simulink model "Non_WindFarm"  (R2024a)
settings: Solver=ode45  StartTime=parSimulacio.ti  StopTime=200  MaxStep=parSimulacio.pas  RelTol=1e-6  AbsTol=1e-6  EnableMultiTasking=on
model workspace (MAT data in the model file):
  tt_vw : Simulink.Parameter (value not decoded)
values from neighbouring files (symbols this model uses):
  L = L'    [Lin_SignalGenerator.m]    (also in Non_ParameterInitialize.m; cal_QR.m = zeros(v, 1); parameters_windFarm2.m)
  nu = size(S, 1)    [Lin_SignalGenerator.m]    (also in Non_ParameterInitialize.m; parameters_windFarm2.m)
  S = zeros(v, v)    [cal_QR.m]
  w0 = [1 -0.00962521549583 0.0254779042049 -0.0160197396127 -0.0156056332727 0.0112137208272 0.0440607583301 -0.0193704893312 -0.0229464276306 -0.00247675309015 0.0285830611299]    [w0.mat]
undefined symbols (not defined in the file or in its folder): parControl, parConvertidor, parGenerador, parGrid, parMecanica, parSimulacio, windspeed
(part 28 of 40)

== system Non_WindFarm/FOM/Wind Farm/Wind Turbine Strings/String6/WT9/WFG/Maquina Sincrona ==
  note: Eq 4.22
  note: park transformation & Inverse
  note: theta_r
  note: Electrical angle=Mechnical angle *Pole Pairs
  note: Omega_r=Omega_m*P
  vsabc : Inport
  omega_m : Inport  Port=2
  theta_m : Inport  Port=3  PortDimensions=1
  Add : Sum  Inputs=+++
  Constant : Constant  Value=-rs/Lq
  Constant1 : Constant  Value=-rs/Ld
  Constant2 : Constant  Value=[1/Lq;0]
  Constant3 : Constant  Value=[1/Lq,0;0,1/Ld]
  Demux : Demux  Outputs=2
  Gain : Gain  Gain=-Ld/Lq
  Gain1 : Gain  Gain=Lq/Ld
  Gain2 : Gain  Gain=-lambda_m
  Gain3 : Gain  Gain=lambda_m
  Gain4 : Gain  Gain=Ld-Lq
  Gain5 : Gain  Gain=3/2*P
  Gain6 : Gain  Gain=P
  Gain7 : Gain  Gain=P
  Integrator : Integrator  InitialCondition=isqd0
  Matrix Concatenate : Concatenate  Mode=Multidimensional array  ConcatenateDimension=2
  Mux : Mux  Inputs=2
  Mux1 : Mux  Inputs=2
  Park : Subsystem
  Product{,2,4..5} (4 alike) : Product  Multiplication=Matrix(*)  RndMeth=Zero
  Product1 : Product  RndMeth=Zero
  Product3 : Product  RndMeth=Zero
  Sum : Sum  Inputs=|++
  isabc : Outport
  parell_m : Outport  Port=2
  wires:
  Constant/1 -> Mux/1
  Gain1/1 -> Mux/2
  Gain/1 -> Mux1/1
  Constant1/1 -> Mux1/2
  omega_m/1 -> Gain6/1
  Mux/1 -> Matrix Concatenate/1
  Mux1/1 -> Matrix Concatenate/2
  Matrix Concatenate/1 -> Product/1
  Product/1 -> Add/1
  Add/1 -> Integrator/1  "disqd"
  Integrator/1 -> Demux/1, Product5/2, Product/2  "isqd"
  Gain2/1 -> Product1/2
  Constant2/1 -> Product1/1
  Product1/1 -> Add/2
  Constant3/1 -> Product2/1
  Product2/1 -> Add/3
  Demux/1 -> Gain3/1, Product3/2
  Product3/1 -> Gain4/1
  Demux/2 -> Product3/1
  Gain3/1 -> Sum/1
  Gain4/1 -> Sum/2
  Sum/1 -> Gain5/1
  Gain5/1 -> parell_m/1
  Gain6/1 -> Gain1/1, Gain/1, Gain2/1
  theta_m/1 -> Gain7/1
  Product4/1 -> Product2/2
  Park/1(Tthetar) -> Product4/1
  Gain7/1 -> Park/1(theta_r)
  Park/2(nTthetar) -> Product5/1
  Product5/1 -> isabc/1
  vsabc/1 -> Product4/2

== system Non_WindFarm/FOM/Wind Farm/Wind Turbine Strings/String6/WT9/WFG/Mecanica nolineal i vent ==
  note: gearbox ration
  note: Gamma_t
  parell_m : Inport
  theta_a : Inport  Port=2
  vw : Inport  Port=3
  Gain1 : Gain  Gain=1/It
  Gain2 : Gain  Gain=nu
  Gain4 : Gain  Gain=nu
  Gain5 : Gain  Gain=nu
  Integrator : Integrator  InitialCondition=omegat0
  Integrator1 : Integrator
  Saturation : Saturate  UpperLimit=inf  LowerLimit=1e-6
  Sum : Sum  Inputs=++|
  Transfer Fcn : TransferFcn  Denominator=[taupitch 1]
  Turbina : Subsystem  mask{rho=1.225, R=R, cs=[0.5 116 0.4 0 0 5 21 0.08 0.035]}
      mask prompts: rho "Densitat de l'aire (Kg/m^3)"; R "Radi (R)"; cs "Constants [c1 c2 .. c9]"
      mask init:
      | A=pi*R^2;
      | c1=cs(1);
      | c2=cs(2);
      | c3=cs(3);
      | c4=cs(4);
      | c5=cs(5);
      | c6=cs(6);
      | c7=cs(7);
      | c8=cs(8);
      | c9=cs(9);
  omega_m : Outport
  theta_m : Outport  Port=2
  Cp : Outport  Port=3
  theta_aleps : Outport  Port=4
  wires:
  Sum/1 -> Gain1/1
  Gain1/1 -> Integrator/1
  Integrator/1 -> Integrator1/1, Gain4/1, Saturation/1
  Turbina/1(parell_turbina) -> Sum/2
  Gain2/1 -> Sum/1
  parell_m/1 -> Gain2/1
  Integrator1/1 -> Gain5/1
  Gain4/1 -> omega_m/1
  Gain5/1 -> theta_m/1
  Saturation/1 -> Turbina/2(omega_aleps)
  Turbina/2(Cp) -> Cp/1
  Transfer Fcn/1 -> theta_aleps/1, Turbina/3(theta_aleps)  "theta_aleps"
  theta_a/1 -> Transfer Fcn/1
  vw/1 -> Turbina/1(velocitat_vent)

== system Non_WindFarm/FOM/Wind Farm/Wind Turbine Strings/String6/WT9/WFG/Park ==
  theta_r : Inport
  Constant4 : Constant  Value=2*pi/3
  Gain7 : Gain  Gain=2/3
  Matrix Concatenate1 : Concatenate  NumInputs=3  Mode=Multidimensional array  ConcatenateDimension=2
  Matrix Concatenate2 : Concatenate  Mode=Multidimensional array  ConcatenateDimension=2
  Mux2 : Mux  Inputs=2
  Mux3 : Mux  Inputs=2
  Mux4 : Mux  Inputs=2
  Mux5 : Mux  Inputs=3
  Mux6 : Mux  Inputs=3
  Sum1 : Sum  Inputs=|++
  Sum2 : Sum  Inputs=|+-
  Trigonometric Function : Trigonometry  Operator=cos
  Trigonometric Function1 : Trigonometry
  Trigonometric Function2 : Trigonometry  Operator=cos
  Trigonometric Function3 : Trigonometry
  Trigonometric Function4 : Trigonometry  Operator=cos
  Trigonometric Function5 : Trigonometry
  Tthetar : Outport
  nTthetar : Outport  Port=2
  wires:
  theta_r/1 -> Sum1/1, Sum2/1, Trigonometric Function/1, Trigonometric Function1/1
  Sum2/1 -> Trigonometric Function2/1, Trigonometric Function3/1
  Sum1/1 -> Trigonometric Function4/1, Trigonometric Function5/1
  Constant4/1 -> Sum2/2, Sum1/2
  Trigonometric Function/1 -> Mux2/1, Mux5/1
  Trigonometric Function1/1 -> Mux2/2, Mux6/1
  Trigonometric Function2/1 -> Mux3/1, Mux5/2
  Trigonometric Function3/1 -> Mux3/2, Mux6/2
  Trigonometric Function4/1 -> Mux4/1, Mux5/3
  Trigonometric Function5/1 -> Mux4/2, Mux6/3
  Mux2/1 -> Matrix Concatenate1/1
  Mux3/1 -> Matrix Concatenate1/2
  Mux4/1 -> Matrix Concatenate1/3
  Matrix Concatenate1/1 -> Gain7/1
  Mux5/1 -> Matrix Concatenate2/1
  Mux6/1 -> Matrix Concatenate2/2
  Gain7/1 -> Tthetar/1
  Matrix Concatenate2/1 -> nTthetar/1

== system Non_WindFarm/FOM/Wind Farm/Wind Turbine Strings/String1/WT1/Transformer-complex/homopolar sequence/Park ==
  theta_r : Inport
  Constant4 : Constant  Value=2*pi/3
  Gain7 : Gain  Gain=2/3
  Matrix Concatenate1 : Concatenate  NumInputs=3  Mode=Multidimensional array  ConcatenateDimension=2
  Matrix Concatenate2 : Concatenate  Mode=Multidimensional array  ConcatenateDimension=2
  Mux2 : Mux  Inputs=2
  Mux3 : Mux  Inputs=2
  Mux4 : Mux  Inputs=2
  Mux5 : Mux  Inputs=3
  Mux6 : Mux  Inputs=3
  Sum1 : Sum  Inputs=|++
  Sum2 : Sum  Inputs=|+-
  Trigonometric Function : Trigonometry  Operator=cos
  Trigonometric Function1 : Trigonometry
  Trigonometric Function2 : Trigonometry  Operator=cos
  Trigonometric Function3 : Trigonometry
  Trigonometric Function4 : Trigonometry  Operator=cos
  Trigonometric Function5 : Trigonometry
  Tthetar : Outport
  nTthetar : Outport  Port=2
  wires:
  theta_r/1 -> Sum1/1, Sum2/1, Trigonometric Function/1, Trigonometric Function1/1
  Sum2/1 -> Trigonometric Function2/1, Trigonometric Function3/1
  Sum1/1 -> Trigonometric Function4/1, Trigonometric Function5/1
  Constant4/1 -> Sum2/2, Sum1/2
  Trigonometric Function/1 -> Mux2/1, Mux5/1
  Trigonometric Function1/1 -> Mux2/2, Mux6/1
  Trigonometric Function2/1 -> Mux3/1, Mux5/2
  Trigonometric Function3/1 -> Mux3/2, Mux6/2
  Trigonometric Function4/1 -> Mux4/1, Mux5/3
  Trigonometric Function5/1 -> Mux4/2, Mux6/3
  Mux2/1 -> Matrix Concatenate1/1
  Mux3/1 -> Matrix Concatenate1/2
  Mux4/1 -> Matrix Concatenate1/3
  Matrix Concatenate1/1 -> Gain7/1
  Mux5/1 -> Matrix Concatenate2/1
  Mux6/1 -> Matrix Concatenate2/2
  Gain7/1 -> Tthetar/1
  Matrix Concatenate2/1 -> nTthetar/1

== system Non_WindFarm/FOM/Wind Farm/Wind Turbine Strings/String1/WT1/Transformer-complex/homopolar sequence/homopolar sequence 1 ==
  note: 1/3*v0
  v : Inport
  Add5 : Sum  Inputs=-+
  Constant : Constant  Value=1/3*ones(3)
  Product3 : Product  Multiplication=Matrix(*)  RndMeth=Zero
  v_bar : Outport
  wires:
  Add5/1 -> v_bar/1
  Product3/1 -> Add5/1
  Constant/1 -> Product3/1
  v/1 -> Product3/2, Add5/2

== system Non_WindFarm/FOM/Wind Farm/Wind Turbine Strings/String1/WT1/Transformer-complex/homopolar sequence/homopolar sequence 2 ==
  note: 1/3*v0
  v : Inport
  Add5 : Sum  Inputs=-+
  Constant : Constant  Value=[1/9,1/9,1/9;1/9,1/9,1/9;1/9,1/9,1/9]
  Product3 : Product  Multiplication=Matrix(*)  RndMeth=Zero
  v_bar : Outport
  wires:
  Add5/1 -> v_bar/1
  Product3/1 -> Add5/1
  Constant/1 -> Product3/1
  v/1 -> Product3/2, Add5/2

== system Non_WindFarm/FOM/Wind Farm/Wind Turbine Strings/String1/WT1/WFG/Control Electric Generador/PI ==
  e : Inport
  Demux : Demux  Outputs=2
  Mux2 : Mux  Inputs=2
  Transfer Fcn : TransferFcn  Numerator=[qKp qKi]  Denominator=[1 0]
  Transfer Fcn1 : TransferFcn  Numerator=[dKp dKi]  Denominator=[1 0]
  u : Outport
  wires:
  Transfer Fcn/1 -> Mux2/1
  Transfer Fcn1/1 -> Mux2/2
  Demux/1 -> Transfer Fcn/1
  Demux/2 -> Transfer Fcn1/1
  e/1 -> Demux/1
  Mux2/1 -> u/1

== system Non_WindFarm/FOM/Wind Farm/Wind Turbine Strings/String1/WT1/WFG/Control Electric Generador/Park ==
  theta_r : Inport
  Constant4 : Constant  Value=2*pi/3
  Gain7 : Gain  Gain=2/3
  Matrix Concatenate1 : Concatenate  NumInputs=3  Mode=Multidimensional array  ConcatenateDimension=2
  Matrix Concatenate2 : Concatenate  Mode=Multidimensional array  ConcatenateDimension=2
  Mux2 : Mux  Inputs=2
  Mux3 : Mux  Inputs=2
  Mux4 : Mux  Inputs=2
  Mux5 : Mux  Inputs=3
  Mux6 : Mux  Inputs=3
  Sum1 : Sum  Inputs=|++
  Sum2 : Sum  Inputs=|+-
  Trigonometric Function : Trigonometry  Operator=cos
  Trigonometric Function1 : Trigonometry
  Trigonometric Function2 : Trigonometry  Operator=cos
  Trigonometric Function3 : Trigonometry
  Trigonometric Function4 : Trigonometry  Operator=cos
  Trigonometric Function5 : Trigonometry
  Tthetar : Outport
  nTthetar : Outport  Port=2
  wires:
  theta_r/1 -> Sum1/1, Sum2/1, Trigonometric Function/1, Trigonometric Function1/1
  Sum2/1 -> Trigonometric Function2/1, Trigonometric Function3/1
  Sum1/1 -> Trigonometric Function4/1, Trigonometric Function5/1
  Constant4/1 -> Sum2/2, Sum1/2
  Trigonometric Function/1 -> Mux2/1, Mux5/1
  Trigonometric Function1/1 -> Mux2/2, Mux6/1
  Trigonometric Function2/1 -> Mux3/1, Mux5/2
  Trigonometric Function3/1 -> Mux3/2, Mux6/2
  Trigonometric Function4/1 -> Mux4/1, Mux5/3
  Trigonometric Function5/1 -> Mux4/2, Mux6/3
  Mux2/1 -> Matrix Concatenate1/1
  Mux3/1 -> Matrix Concatenate1/2
  Mux4/1 -> Matrix Concatenate1/3
  Matrix Concatenate1/1 -> Gain7/1
  Mux5/1 -> Matrix Concatenate2/1
  Mux6/1 -> Matrix Concatenate2/2
  Gain7/1 -> Tthetar/1
  Matrix Concatenate2/1 -> nTthetar/1

== system Non_WindFarm/FOM/Wind Farm/Wind Turbine Strings/String1/WT1/WFG/Control Electric Generador/Sat inf ==
  in : Inport
  Abs : Abs  SaturateOnIntegerOverflow=off
  Constant3 : Constant  Value=0.01
  Relational Operator : RelationalOperator  Operator=>  OutDataTypeStr=boolean  InputSameDT=off
  Switch : Switch  Criteria=u2 > Threshold  SaturateOnIntegerOverflow=off  InputSameDT=off
  out : Outport
  wires:
  Abs/1 -> Relational Operator/1
  Constant3/1 -> Relational Operator/2, Switch/3
  Relational Operator/1 -> Switch/2
  in/1 -> Abs/1, Switch/1
  Switch/1 -> out/1

== system Non_WindFarm/FOM/Wind Farm/Wind Turbine Strings/String1/WT1/WFG/Control de Corrent de Xarxa2/PI_d ==
  e : Inport
  Demux : Demux  Outputs=2
  Mux2 : Mux  Inputs=2
  Transfer Fcn : TransferFcn  Numerator=[Kp Ki]  Denominator=[1,0]
  Transfer Fcn1 : TransferFcn  Numerator=[Kp Ki]  Denominator=[1,0]
  u : Outport
  wires:
  Transfer Fcn/1 -> Mux2/1
  Transfer Fcn1/1 -> Mux2/2
  Demux/1 -> Transfer Fcn/1
  Demux/2 -> Transfer Fcn1/1
  e/1 -> Demux/1
  Mux2/1 -> u/1

== system Non_WindFarm/FOM/Wind Farm/Wind Turbine Strings/String1/WT1/WFG/Control de Corrent de Xarxa2/rotacio1 ==
  theta : Inport
  Constant1 : Constant  Value=2*pi/3
  Gain1 : Gain  Gain=-1
  Matrix Concatenate1 : Concatenate  Mode=Multidimensional array  ConcatenateDimension=2
  Matrix Concatenate2 : Concatenate  Mode=Multidimensional array  ConcatenateDimension=2
  Mux1 : Mux  Inputs=3
  Mux2 : Mux  Inputs=2
  Mux3 : Mux  Inputs=2
  Mux5 : Mux  Inputs=3
  Sum4 : Sum  Inputs=|+-
  Sum5 : Sum  Inputs=|++
  Sum6 : Sum  Inputs=|+-
  Sum7 : Sum  Inputs=|++
  Trigonometric Function{,6,8,10} (4 alike) : Trigonometry  Operator=cos
  Trigonometric Function{1,7,9,11} (4 alike) : Trigonometry
  T : Outport
  nT : Outport  Port=2
  wires:
  Trigonometric Function/1 -> Mux2/1, Mux3/2
  Trigonometric Function1/1 -> Gain1/1, Mux2/2
  Mux2/1 -> Matrix Concatenate1/1
  Mux3/1 -> Matrix Concatenate1/2
  Matrix Concatenate1/1 -> T/1
  Matrix Concatenate2/1 -> nT/1
  theta/1 -> Trigonometric Function6/1, Sum4/1, Sum5/1, Trigonometric Function9/1, Sum6/1, Sum7/1, Trigonometric Function/1, Trigonometric Function1/1
  Sum4/1 -> Trigonometric Function10/1
  Constant1/1 -> Sum4/2, Sum5/2, Sum6/2, Sum7/2
  Sum5/1 -> Trigonometric Function8/1
  Sum6/1 -> Trigonometric Function7/1
  Sum7/1 -> Trigonometric Function11/1
  Trigonometric Function6/1 -> Mux5/1
  Trigonometric Function10/1 -> Mux5/2
  Trigonometric Function8/1 -> Mux5/3
  Trigonometric Function9/1 -> Mux1/1
  Trigonometric Function7/1 -> Mux1/2
  Trigonometric Function11/1 -> Mux1/3
  Mux5/1 -> Matrix Concatenate2/1
  Mux1/1 -> Matrix Concatenate2/2
  Gain1/1 -> Mux3/1

== system Non_WindFarm/FOM/Wind Farm/Wind Turbine Strings/String1/WT1/WFG/Maquina Sincrona/Park ==
  note: Page 24 eq 3.12
  theta_r : Inport
  Constant4 : Constant  Value=2*pi/3
  Gain7 : Gain  Gain=2/3
  Matrix Concatenate1 : Concatenate  NumInputs=3  Mode=Multidimensional array  ConcatenateDimension=2
  Matrix Concatenate2 : Concatenate  Mode=Multidimensional array  ConcatenateDimension=2
  Mux2 : Mux  Inputs=2
  Mux3 : Mux  Inputs=2
  Mux4 : Mux  Inputs=2
  Mux5 : Mux  Inputs=3
  Mux6 : Mux  Inputs=3
  Sum1 : Sum  Inputs=|++
  Sum2 : Sum  Inputs=|+-
  Trigonometric Function : Trigonometry  Operator=cos
  Trigonometric Function1 : Trigonometry
  Trigonometric Function2 : Trigonometry  Operator=cos
  Trigonometric Function3 : Trigonometry
  Trigonometric Function4 : Trigonometry  Operator=cos
  Trigonometric Function5 : Trigonometry
  Tthetar : Outport
  nTthetar : Outport  Port=2
  wires:
  Constant4/1 -> Sum2/2, Sum1/2
  Trigonometric Function/1 -> Mux2/1, Mux5/1
  Trigonometric Function1/1 -> Mux2/2, Mux6/1
  Trigonometric Function2/1 -> Mux3/1, Mux5/2
  Trigonometric Function3/1 -> Mux3/2, Mux6/2
  Trigonometric Function4/1 -> Mux4/1, Mux5/3
  Trigonometric Function5/1 -> Mux4/2, Mux6/3
  Mux2/1 -> Matrix Concatenate1/1
  Mux3/1 -> Matrix Concatenate1/2
  Mux4/1 -> Matrix Concatenate1/3
  Matrix Concatenate1/1 -> Gain7/1
  Mux5/1 -> Matrix Concatenate2/1
  Mux6/1 -> Matrix Concatenate2/2
  Gain7/1 -> Tthetar/1
  Matrix Concatenate2/1 -> nTthetar/1
  theta_r/1 -> Sum1/1, Sum2/1, Trigonometric Function1/1, Trigonometric Function/1
  Sum2/1 -> Trigonometric Function3/1, Trigonometric Function2/1
  Sum1/1 -> Trigonometric Function5/1, Trigonometric Function4/1

== system Non_WindFarm/FOM/Wind Farm/Wind Turbine Strings/String1/WT1/WFG/Mecanica nolineal i vent/Turbina ==
  note: Page 8
  note: Gamma_t-Wind turbine torque
  note: Wt-turbine speed
  note: Vw-wind speed
  note: Beta-pitch angle
  velocitat_vent : Inport
  omega_aleps : Inport  Port=2
  theta_aleps : Inport  Port=3
  Calcula_Cp : Fcn  Expr=c1*(c2*u[1]-c3*u[2]-c4*u[2]^c5-c6)*exp(-c7*u[1])
  Calcula_parell : Fcn  Expr=u[1]*rho*A*u[2]^3/(2*u[3])
  LAMBDA_inversa : Fcn  Expr=1/(u[1]+c8*u[2])-c9/(1+u[2]^3)
  Mux : Mux  Inputs=2
  Mux1 : Mux  Inputs=2
  Mux2 : Mux  Inputs=2
  Mux3 : Mux  Inputs=3
  calcula_lambda : Fcn  Expr=u[2]*R/u[1]
  parell_turbina : Outport
  Cp : Outport  Port=2
  wires:
  Mux1/1 -> calcula_lambda/1
  omega_aleps/1 -> Mux1/2, Mux3/3
  velocitat_vent/1 -> Mux1/1, Mux3/2
  calcula_lambda/1 -> Mux/1
  theta_aleps/1 -> Mux/2, Mux2/2
  Mux/1 -> LAMBDA_inversa/1
  LAMBDA_inversa/1 -> Mux2/1
  Mux2/1 -> Calcula_Cp/1
  Calcula_Cp/1 -> Mux3/1, Cp/1
  Mux3/1 -> Calcula_parell/1
  Calcula_parell/1 -> parell_turbina/1

== system Non_WindFarm/FOM/Wind Farm/Wind Turbine Strings/String1/WT10/Transformer-complex/homopolar sequence/Park ==
  theta_r : Inport
  Constant4 : Constant  Value=2*pi/3
  Gain7 : Gain  Gain=2/3
  Matrix Concatenate1 : Concatenate  NumInputs=3  Mode=Multidimensional array  ConcatenateDimension=2
  Matrix Concatenate2 : Concatenate  Mode=Multidimensional array  ConcatenateDimension=2
  Mux2 : Mux  Inputs=2
  Mux3 : Mux  Inputs=2
  Mux4 : Mux  Inputs=2
  Mux5 : Mux  Inputs=3
  Mux6 : Mux  Inputs=3
  Sum1 : Sum  Inputs=|++
  Sum2 : Sum  Inputs=|+-
  Trigonometric Function : Trigonometry  Operator=cos
  Trigonometric Function1 : Trigonometry
  Trigonometric Function2 : Trigonometry  Operator=cos
  Trigonometric Function3 : Trigonometry
  Trigonometric Function4 : Trigonometry  Operator=cos
  Trigonometric Function5 : Trigonometry
  Tthetar : Outport
  nTthetar : Outport  Port=2
  wires:
  Matrix Concatenate2/1 -> nTthetar/1
  Gain7/1 -> Tthetar/1
  Mux6/1 -> Matrix Concatenate2/2
  Mux5/1 -> Matrix Concatenate2/1
  Matrix Concatenate1/1 -> Gain7/1
  Mux4/1 -> Matrix Concatenate1/3
  Mux3/1 -> Matrix Concatenate1/2
  Mux2/1 -> Matrix Concatenate1/1
  Trigonometric Function5/1 -> Mux6/3, Mux4/2
  Trigonometric Function4/1 -> Mux5/3, Mux4/1
  Trigonometric Function3/1 -> Mux6/2, Mux3/2
  Trigonometric Function2/1 -> Mux5/2, Mux3/1
  Trigonometric Function1/1 -> Mux6/1, Mux2/2
  Trigonometric Function/1 -> Mux5/1, Mux2/1
  Constant4/1 -> Sum1/2, Sum2/2
  Sum1/1 -> Trigonometric Function5/1, Trigonometric Function4/1
  Sum2/1 -> Trigonometric Function3/1, Trigonometric Function2/1
  theta_r/1 -> Trigonometric Function1/1, Trigonometric Function/1, Sum2/1, Sum1/1

== system Non_WindFarm/FOM/Wind Farm/Wind Turbine Strings/String1/WT10/Transformer-complex/homopolar sequence/homopolar sequence 1 ==
  note: 1/3*v0
  v : Inport
  Add5 : Sum  Inputs=-+
  Constant : Constant  Value=1/3*ones(3)
  Product3 : Product  Multiplication=Matrix(*)  RndMeth=Zero
  v_bar : Outport
  wires:
  v/1 -> Add5/2, Product3/2
  Constant/1 -> Product3/1
  Product3/1 -> Add5/1
  Add5/1 -> v_bar/1

== system Non_WindFarm/FOM/Wind Farm/Wind Turbine Strings/String1/WT10/Transformer-complex/homopolar sequence/homopolar sequence 2 ==
  note: 1/3*v0
  v : Inport
  Add5 : Sum  Inputs=-+
  Constant : Constant  Value=[1/9,1/9,1/9;1/9,1/9,1/9;1/9,1/9,1/9]
  Product3 : Product  Multiplication=Matrix(*)  RndMeth=Zero
  v_bar : Outport
  wires:
  v/1 -> Add5/2, Product3/2
  Constant/1 -> Product3/1
  Product3/1 -> Add5/1
  Add5/1 -> v_bar/1

== system Non_WindFarm/FOM/Wind Farm/Wind Turbine Strings/String1/WT10/WFG/Control Electric Generador/PI ==
  e : Inport
  Demux : Demux  Outputs=2
  Mux2 : Mux  Inputs=2
  Transfer Fcn : TransferFcn  Numerator=[qKp qKi]  Denominator=[1 0]
  Transfer Fcn1 : TransferFcn  Numerator=[dKp dKi]  Denominator=[1 0]
  u : Outport
  wires:
  Mux2/1 -> u/1
  e/1 -> Demux/1
  Demux/2 -> Transfer Fcn1/1
  Demux/1 -> Transfer Fcn/1
  Transfer Fcn1/1 -> Mux2/2
  Transfer Fcn/1 -> Mux2/1

== system Non_WindFarm/FOM/Wind Farm/Wind Turbine Strings/String1/WT10/WFG/Control Electric Generador/Park ==
  theta_r : Inport
  Constant4 : Constant  Value=2*pi/3
  Gain7 : Gain  Gain=2/3
  Matrix Concatenate1 : Concatenate  NumInputs=3  Mode=Multidimensional array  ConcatenateDimension=2
  Matrix Concatenate2 : Concatenate  Mode=Multidimensional array  ConcatenateDimension=2
  Mux2 : Mux  Inputs=2
  Mux3 : Mux  Inputs=2
  Mux4 : Mux  Inputs=2
  Mux5 : Mux  Inputs=3
  Mux6 : Mux  Inputs=3
  Sum1 : Sum  Inputs=|++
  Sum2 : Sum  Inputs=|+-
  Trigonometric Function : Trigonometry  Operator=cos
  Trigonometric Function1 : Trigonometry
  Trigonometric Function2 : Trigonometry  Operator=cos
  Trigonometric Function3 : Trigonometry
  Trigonometric Function4 : Trigonometry  Operator=cos
  Trigonometric Function5 : Trigonometry
  Tthetar : Outport
  nTthetar : Outport  Port=2
  wires:
  Matrix Concatenate2/1 -> nTthetar/1
  Gain7/1 -> Tthetar/1
  Mux6/1 -> Matrix Concatenate2/2
  Mux5/1 -> Matrix Concatenate2/1
  Matrix Concatenate1/1 -> Gain7/1
  Mux4/1 -> Matrix Concatenate1/3
  Mux3/1 -> Matrix Concatenate1/2
  Mux2/1 -> Matrix Concatenate1/1
  Trigonometric Function5/1 -> Mux6/3, Mux4/2
  Trigonometric Function4/1 -> Mux5/3, Mux4/1
  Trigonometric Function3/1 -> Mux6/2, Mux3/2
  Trigonometric Function2/1 -> Mux5/2, Mux3/1
  Trigonometric Function1/1 -> Mux6/1, Mux2/2
  Trigonometric Function/1 -> Mux5/1, Mux2/1
  Constant4/1 -> Sum1/2, Sum2/2
  Sum1/1 -> Trigonometric Function5/1, Trigonometric Function4/1
  Sum2/1 -> Trigonometric Function3/1, Trigonometric Function2/1
  theta_r/1 -> Trigonometric Function1/1, Trigonometric Function/1, Sum2/1, Sum1/1

== system Non_WindFarm/FOM/Wind Farm/Wind Turbine Strings/String1/WT10/WFG/Control Electric Generador/Sat inf ==
  in : Inport
  Abs : Abs  SaturateOnIntegerOverflow=off
  Constant3 : Constant  Value=0.01
  Relational Operator : RelationalOperator  Operator=>  OutDataTypeStr=boolean  InputSameDT=off
  Switch : Switch  Criteria=u2 > Threshold  SaturateOnIntegerOverflow=off  InputSameDT=off
  out : Outport
  wires:
  Switch/1 -> out/1
  in/1 -> Switch/1, Abs/1
  Relational Operator/1 -> Switch/2
  Constant3/1 -> Switch/3, Relational Operator/2
  Abs/1 -> Relational Operator/1

== system Non_WindFarm/FOM/Wind Farm/Wind Turbine Strings/String1/WT10/WFG/Control de Corrent de Xarxa2/PI_d ==
  e : Inport
  Demux : Demux  Outputs=2
  Mux2 : Mux  Inputs=2
  Transfer Fcn : TransferFcn  Numerator=[Kp Ki]  Denominator=[1,0]
  Transfer Fcn1 : TransferFcn  Numerator=[Kp Ki]  Denominator=[1,0]
  u : Outport
  wires:
  Mux2/1 -> u/1
  e/1 -> Demux/1
  Demux/2 -> Transfer Fcn1/1
  Demux/1 -> Transfer Fcn/1
  Transfer Fcn1/1 -> Mux2/2
  Transfer Fcn/1 -> Mux2/1

== system Non_WindFarm/FOM/Wind Farm/Wind Turbine Strings/String1/WT10/WFG/Control de Corrent de Xarxa2/rotacio1 ==
  theta : Inport
  Constant1 : Constant  Value=2*pi/3
  Gain1 : Gain  Gain=-1
  Matrix Concatenate1 : Concatenate  Mode=Multidimensional array  ConcatenateDimension=2
  Matrix Concatenate2 : Concatenate  Mode=Multidimensional array  ConcatenateDimension=2
  Mux1 : Mux  Inputs=3
  Mux2 : Mux  Inputs=2
  Mux3 : Mux  Inputs=2
  Mux5 : Mux  Inputs=3
  Sum4 : Sum  Inputs=|+-
  Sum5 : Sum  Inputs=|++
  Sum6 : Sum  Inputs=|+-
  Sum7 : Sum  Inputs=|++
  Trigonometric Function{,6,8,10} (4 alike) : Trigonometry  Operator=cos
  Trigonometric Function{1,7,9,11} (4 alike) : Trigonometry
  T : Outport
  nT : Outport  Port=2
  wires:
  Gain1/1 -> Mux3/1
  Mux1/1 -> Matrix Concatenate2/2
  Mux5/1 -> Matrix Concatenate2/1
  Trigonometric Function11/1 -> Mux1/3
  Trigonometric Function7/1 -> Mux1/2
  Trigonometric Function9/1 -> Mux1/1
  Trigonometric Function8/1 -> Mux5/3
  Trigonometric Function10/1 -> Mux5/2
  Trigonometric Function6/1 -> Mux5/1
  Sum7/1 -> Trigonometric Function11/1
  Sum6/1 -> Trigonometric Function7/1
  Sum5/1 -> Trigonometric Function8/1
  Constant1/1 -> Sum7/2, Sum6/2, Sum5/2, Sum4/2
  Sum4/1 -> Trigonometric Function10/1
  theta/1 -> Trigonometric Function1/1, Trigonometric Function/1, Sum7/1, Sum6/1, Trigonometric Function9/1, Sum5/1, Sum4/1, Trigonometric Function6/1
  Matrix Concatenate2/1 -> nT/1
  Matrix Concatenate1/1 -> T/1
  Mux3/1 -> Matrix Concatenate1/2
  Mux2/1 -> Matrix Concatenate1/1
  Trigonometric Function1/1 -> Mux2/2, Gain1/1
  Trigonometric Function/1 -> Mux3/2, Mux2/1

== system Non_WindFarm/FOM/Wind Farm/Wind Turbine Strings/String1/WT10/WFG/Maquina Sincrona/Park ==
  note: Page 24 eq 3.12
  theta_r : Inport
  Constant4 : Constant  Value=2*pi/3
  Gain7 : Gain  Gain=2/3
  Matrix Concatenate1 : Concatenate  NumInputs=3  Mode=Multidimensional array  ConcatenateDimension=2
  Matrix Concatenate2 : Concatenate  Mode=Multidimensional array  ConcatenateDimension=2
  Mux2 : Mux  Inputs=2
  Mux3 : Mux  Inputs=2
  Mux4 : Mux  Inputs=2
  Mux5 : Mux  Inputs=3
  Mux6 : Mux  Inputs=3
  Sum1 : Sum  Inputs=|++
  Sum2 : Sum  Inputs=|+-
  Trigonometric Function : Trigonometry  Operator=cos
  Trigonometric Function1 : Trigonometry
  Trigonometric Function2 : Trigonometry  Operator=cos
  Trigonometric Function3 : Trigonometry
  Trigonometric Function4 : Trigonometry  Operator=cos
  Trigonometric Function5 : Trigonometry
  Tthetar : Outport
  nTthetar : Outport  Port=2
  wires:
  Sum1/1 -> Trigonometric Function4/1, Trigonometric Function5/1
  Sum2/1 -> Trigonometric Function2/1, Trigonometric Function3/1
  theta_r/1 -> Trigonometric Function/1, Trigonometric Function1/1, Sum2/1, Sum1/1
  Matrix Concatenate2/1 -> nTthetar/1
  Gain7/1 -> Tthetar/1
  Mux6/1 -> Matrix Concatenate2/2
  Mux5/1 -> Matrix Concatenate2/1
  Matrix Concatenate1/1 -> Gain7/1
  Mux4/1 -> Matrix Concatenate1/3
  Mux3/1 -> Matrix Concatenate1/2
  Mux2/1 -> Matrix Concatenate1/1
  Trigonometric Function5/1 -> Mux6/3, Mux4/2
  Trigonometric Function4/1 -> Mux5/3, Mux4/1
  Trigonometric Function3/1 -> Mux6/2, Mux3/2
  Trigonometric Function2/1 -> Mux5/2, Mux3/1
  Trigonometric Function1/1 -> Mux6/1, Mux2/2
  Trigonometric Function/1 -> Mux5/1, Mux2/1
  Constant4/1 -> Sum1/2, Sum2/2

== system Non_WindFarm/FOM/Wind Farm/Wind Turbine Strings/String1/WT10/WFG/Mecanica nolineal i vent/Turbina ==
  note: Beta-pitch angle
  note: Vw-wind speed
  note: Wt-turbine speed
  note: Gamma_t-Wind turbine torque
  note: Page 8
  velocitat_vent : Inport
  omega_aleps : Inport  Port=2
  theta_aleps : Inport  Port=3
  Calcula_Cp : Fcn  Expr=c1*(c2*u[1]-c3*u[2]-c4*u[2]^c5-c6)*exp(-c7*u[1])
  Calcula_parell : Fcn  Expr=u[1]*rho*A*u[2]^3/(2*u[3])
  LAMBDA_inversa : Fcn  Expr=1/(u[1]+c8*u[2])-c9/(1+u[2]^3)
  Mux : Mux  Inputs=2
  Mux1 : Mux  Inputs=2
  Mux2 : Mux  Inputs=2
  Mux3 : Mux  Inputs=3
  calcula_lambda : Fcn  Expr=u[2]*R/u[1]
  parell_turbina : Outport
  Cp : Outport  Port=2
  wires:
  Calcula_parell/1 -> parell_turbina/1
  Mux3/1 -> Calcula_parell/1
  Calcula_Cp/1 -> Cp/1, Mux3/1
  Mux2/1 -> Calcula_Cp/1
  LAMBDA_inversa/1 -> Mux2/1
  Mux/1 -> LAMBDA_inversa/1
  theta_aleps/1 -> Mux2/2, Mux/2
  calcula_lambda/1 -> Mux/1
  velocitat_vent/1 -> Mux3/2, Mux1/1
  omega_aleps/1 -> Mux3/3, Mux1/2
  Mux1/1 -> calcula_lambda/1

== system Non_WindFarm/FOM/Wind Farm/Wind Turbine Strings/String1/WT2/Transformer-complex/homopolar sequence/Park ==
  theta_r : Inport
  Constant4 : Constant  Value=2*pi/3
  Gain7 : Gain  Gain=2/3
  Matrix Concatenate1 : Concatenate  NumInputs=3  Mode=Multidimensional array  ConcatenateDimension=2
  Matrix Concatenate2 : Concatenate  Mode=Multidimensional array  ConcatenateDimension=2
  Mux2 : Mux  Inputs=2
  Mux3 : Mux  Inputs=2
  Mux4 : Mux  Inputs=2
  Mux5 : Mux  Inputs=3
  Mux6 : Mux  Inputs=3
  Sum1 : Sum  Inputs=|++
  Sum2 : Sum  Inputs=|+-
  Trigonometric Function : Trigonometry  Operator=cos
  Trigonometric Function1 : Trigonometry
  Trigonometric Function2 : Trigonometry  Operator=cos
  Trigonometric Function3 : Trigonometry
  Trigonometric Function4 : Trigonometry  Operator=cos
  Trigonometric Function5 : Trigonometry
  Tthetar : Outport
  nTthetar : Outport  Port=2
  wires:
  Matrix Concatenate2/1 -> nTthetar/1
  Gain7/1 -> Tthetar/1
  Mux6/1 -> Matrix Concatenate2/2
  Mux5/1 -> Matrix Concatenate2/1
  Matrix Concatenate1/1 -> Gain7/1
  Mux4/1 -> Matrix Concatenate1/3
  Mux3/1 -> Matrix Concatenate1/2
  Mux2/1 -> Matrix Concatenate1/1
  Trigonometric Function5/1 -> Mux6/3, Mux4/2
  Trigonometric Function4/1 -> Mux5/3, Mux4/1
  Trigonometric Function3/1 -> Mux6/2, Mux3/2
  Trigonometric Function2/1 -> Mux5/2, Mux3/1
  Trigonometric Function1/1 -> Mux6/1, Mux2/2
  Trigonometric Function/1 -> Mux5/1, Mux2/1
  Constant4/1 -> Sum1/2, Sum2/2
  Sum1/1 -> Trigonometric Function5/1, Trigonometric Function4/1
  Sum2/1 -> Trigonometric Function3/1, Trigonometric Function2/1
  theta_r/1 -> Trigonometric Function1/1, Trigonometric Function/1, Sum2/1, Sum1/1

== system Non_WindFarm/FOM/Wind Farm/Wind Turbine Strings/String1/WT2/Transformer-complex/homopolar sequence/homopolar sequence 1 ==
  note: 1/3*v0
  v : Inport
  Add5 : Sum  Inputs=-+
  Constant : Constant  Value=1/3*ones(3)
  Product3 : Product  Multiplication=Matrix(*)  RndMeth=Zero
  v_bar : Outport
  wires:
  v/1 -> Add5/2, Product3/2
  Constant/1 -> Product3/1
  Product3/1 -> Add5/1
  Add5/1 -> v_bar/1

== system Non_WindFarm/FOM/Wind Farm/Wind Turbine Strings/String1/WT2/Transformer-complex/homopolar sequence/homopolar sequence 2 ==
  note: 1/3*v0
  v : Inport
  Add5 : Sum  Inputs=-+
  Constant : Constant  Value=[1/9,1/9,1/9;1/9,1/9,1/9;1/9,1/9,1/9]
  Product3 : Product  Multiplication=Matrix(*)  RndMeth=Zero
  v_bar : Outport
  wires:
  v/1 -> Add5/2, Product3/2
  Constant/1 -> Product3/1
  Product3/1 -> Add5/1
  Add5/1 -> v_bar/1

== system Non_WindFarm/FOM/Wind Farm/Wind Turbine Strings/String1/WT2/WFG/Control Electric Generador/PI ==
  e : Inport
  Demux : Demux  Outputs=2
  Mux2 : Mux  Inputs=2
  Transfer Fcn : TransferFcn  Numerator=[qKp qKi]  Denominator=[1 0]
  Transfer Fcn1 : TransferFcn  Numerator=[dKp dKi]  Denominator=[1 0]
  u : Outport
  wires:
  Mux2/1 -> u/1
  e/1 -> Demux/1
  Demux/2 -> Transfer Fcn1/1
  Demux/1 -> Transfer Fcn/1
  Transfer Fcn1/1 -> Mux2/2
  Transfer Fcn/1 -> Mux2/1

== system Non_WindFarm/FOM/Wind Farm/Wind Turbine Strings/String1/WT2/WFG/Control Electric Generador/Park ==
  theta_r : Inport
  Constant4 : Constant  Value=2*pi/3
  Gain7 : Gain  Gain=2/3
  Matrix Concatenate1 : Concatenate  NumInputs=3  Mode=Multidimensional array  ConcatenateDimension=2
  Matrix Concatenate2 : Concatenate  Mode=Multidimensional array  ConcatenateDimension=2
  Mux2 : Mux  Inputs=2
  Mux3 : Mux  Inputs=2
  Mux4 : Mux  Inputs=2
  Mux5 : Mux  Inputs=3
  Mux6 : Mux  Inputs=3
  Sum1 : Sum  Inputs=|++
  Sum2 : Sum  Inputs=|+-
  Trigonometric Function : Trigonometry  Operator=cos
  Trigonometric Function1 : Trigonometry
  Trigonometric Function2 : Trigonometry  Operator=cos
  Trigonometric Function3 : Trigonometry
  Trigonometric Function4 : Trigonometry  Operator=cos
  Trigonometric Function5 : Trigonometry
  Tthetar : Outport
  nTthetar : Outport  Port=2
  wires:
  Matrix Concatenate2/1 -> nTthetar/1
  Gain7/1 -> Tthetar/1
  Mux6/1 -> Matrix Concatenate2/2
  Mux5/1 -> Matrix Concatenate2/1
  Matrix Concatenate1/1 -> Gain7/1
  Mux4/1 -> Matrix Concatenate1/3
  Mux3/1 -> Matrix Concatenate1/2
  Mux2/1 -> Matrix Concatenate1/1
  Trigonometric Function5/1 -> Mux6/3, Mux4/2
  Trigonometric Function4/1 -> Mux5/3, Mux4/1
  Trigonometric Function3/1 -> Mux6/2, Mux3/2
  Trigonometric Function2/1 -> Mux5/2, Mux3/1
  Trigonometric Function1/1 -> Mux6/1, Mux2/2
  Trigonometric Function/1 -> Mux5/1, Mux2/1
  Constant4/1 -> Sum1/2, Sum2/2
  Sum1/1 -> Trigonometric Function5/1, Trigonometric Function4/1
  Sum2/1 -> Trigonometric Function3/1, Trigonometric Function2/1
  theta_r/1 -> Trigonometric Function1/1, Trigonometric Function/1, Sum2/1, Sum1/1

== system Non_WindFarm/FOM/Wind Farm/Wind Turbine Strings/String1/WT2/WFG/Control Electric Generador/Sat inf ==
  in : Inport
  Abs : Abs  SaturateOnIntegerOverflow=off
  Constant3 : Constant  Value=0.01
  Relational Operator : RelationalOperator  Operator=>  OutDataTypeStr=boolean  InputSameDT=off
  Switch : Switch  Criteria=u2 > Threshold  SaturateOnIntegerOverflow=off  InputSameDT=off
  out : Outport
  wires:
  Switch/1 -> out/1
  in/1 -> Switch/1, Abs/1
  Relational Operator/1 -> Switch/2
  Constant3/1 -> Switch/3, Relational Operator/2
  Abs/1 -> Relational Operator/1

== system Non_WindFarm/FOM/Wind Farm/Wind Turbine Strings/String1/WT2/WFG/Control de Corrent de Xarxa2/PI_d ==
  e : Inport
  Demux : Demux  Outputs=2
  Mux2 : Mux  Inputs=2
  Transfer Fcn : TransferFcn  Numerator=[Kp Ki]  Denominator=[1,0]
  Transfer Fcn1 : TransferFcn  Numerator=[Kp Ki]  Denominator=[1,0]
  u : Outport
  wires:
  Mux2/1 -> u/1
  e/1 -> Demux/1
  Demux/2 -> Transfer Fcn1/1
  Demux/1 -> Transfer Fcn/1
  Transfer Fcn1/1 -> Mux2/2
  Transfer Fcn/1 -> Mux2/1

== system Non_WindFarm/FOM/Wind Farm/Wind Turbine Strings/String1/WT2/WFG/Control de Corrent de Xarxa2/rotacio1 ==
  theta : Inport
  Constant1 : Constant  Value=2*pi/3
  Gain1 : Gain  Gain=-1
  Matrix Concatenate1 : Concatenate  Mode=Multidimensional array  ConcatenateDimension=2
  Matrix Concatenate2 : Concatenate  Mode=Multidimensional array  ConcatenateDimension=2
  Mux1 : Mux  Inputs=3
  Mux2 : Mux  Inputs=2
  Mux3 : Mux  Inputs=2
  Mux5 : Mux  Inputs=3
  Sum4 : Sum  Inputs=|+-
  Sum5 : Sum  Inputs=|++
  Sum6 : Sum  Inputs=|+-
  Sum7 : Sum  Inputs=|++
  Trigonometric Function{,6,8,10} (4 alike) : Trigonometry  Operator=cos
  Trigonometric Function{1,7,9,11} (4 alike) : Trigonometry
  T : Outport
  nT : Outport  Port=2
  wires:
  Gain1/1 -> Mux3/1
  Mux1/1 -> Matrix Concatenate2/2
  Mux5/1 -> Matrix Concatenate2/1
  Trigonometric Function11/1 -> Mux1/3
  Trigonometric Function7/1 -> Mux1/2
  Trigonometric Function9/1 -> Mux1/1
  Trigonometric Function8/1 -> Mux5/3
  Trigonometric Function10/1 -> Mux5/2
  Trigonometric Function6/1 -> Mux5/1
  Sum7/1 -> Trigonometric Function11/1
  Sum6/1 -> Trigonometric Function7/1
  Sum5/1 -> Trigonometric Function8/1
  Constant1/1 -> Sum7/2, Sum6/2, Sum5/2, Sum4/2
  Sum4/1 -> Trigonometric Function10/1
  theta/1 -> Trigonometric Function1/1, Trigonometric Function/1, Sum7/1, Sum6/1, Trigonometric Function9/1, Sum5/1, Sum4/1, Trigonometric Function6/1
  Matrix Concatenate2/1 -> nT/1
  Matrix Concatenate1/1 -> T/1
  Mux3/1 -> Matrix Concatenate1/2
  Mux2/1 -> Matrix Concatenate1/1
  Trigonometric Function1/1 -> Mux2/2, Gain1/1
  Trigonometric Function/1 -> Mux3/2, Mux2/1

== system Non_WindFarm/FOM/Wind Farm/Wind Turbine Strings/String1/WT2/WFG/Maquina Sincrona/Park ==
  note: Page 24 eq 3.12
  theta_r : Inport
  Constant4 : Constant  Value=2*pi/3
  Gain7 : Gain  Gain=2/3
  Matrix Concatenate1 : Concatenate  NumInputs=3  Mode=Multidimensional array  ConcatenateDimension=2
  Matrix Concatenate2 : Concatenate  Mode=Multidimensional array  ConcatenateDimension=2
  Mux2 : Mux  Inputs=2
  Mux3 : Mux  Inputs=2
  Mux4 : Mux  Inputs=2
  Mux5 : Mux  Inputs=3
  Mux6 : Mux  Inputs=3
  Sum1 : Sum  Inputs=|++
  Sum2 : Sum  Inputs=|+-
  Trigonometric Function : Trigonometry  Operator=cos
  Trigonometric Function1 : Trigonometry
  Trigonometric Function2 : Trigonometry  Operator=cos
  Trigonometric Function3 : Trigonometry
  Trigonometric Function4 : Trigonometry  Operator=cos
  Trigonometric Function5 : Trigonometry
  Tthetar : Outport
  nTthetar : Outport  Port=2
  wires:
  Sum1/1 -> Trigonometric Function4/1, Trigonometric Function5/1
  Sum2/1 -> Trigonometric Function2/1, Trigonometric Function3/1
  theta_r/1 -> Trigonometric Function/1, Trigonometric Function1/1, Sum2/1, Sum1/1
  Matrix Concatenate2/1 -> nTthetar/1
  Gain7/1 -> Tthetar/1
  Mux6/1 -> Matrix Concatenate2/2
  Mux5/1 -> Matrix Concatenate2/1
  Matrix Concatenate1/1 -> Gain7/1
  Mux4/1 -> Matrix Concatenate1/3
  Mux3/1 -> Matrix Concatenate1/2
  Mux2/1 -> Matrix Concatenate1/1
  Trigonometric Function5/1 -> Mux6/3, Mux4/2
  Trigonometric Function4/1 -> Mux5/3, Mux4/1
  Trigonometric Function3/1 -> Mux6/2, Mux3/2
  Trigonometric Function2/1 -> Mux5/2, Mux3/1
  Trigonometric Function1/1 -> Mux6/1, Mux2/2
  Trigonometric Function/1 -> Mux5/1, Mux2/1
  Constant4/1 -> Sum1/2, Sum2/2

== system Non_WindFarm/FOM/Wind Farm/Wind Turbine Strings/String1/WT2/WFG/Mecanica nolineal i vent/Turbina ==
  note: Beta-pitch angle
  note: Vw-wind speed
  note: Wt-turbine speed
  note: Gamma_t-Wind turbine torque
  note: Page 8
  velocitat_vent : Inport
  omega_aleps : Inport  Port=2
  theta_aleps : Inport  Port=3
  Calcula_Cp : Fcn  Expr=c1*(c2*u[1]-c3*u[2]-c4*u[2]^c5-c6)*exp(-c7*u[1])
  Calcula_parell : Fcn  Expr=u[1]*rho*A*u[2]^3/(2*u[3])
  LAMBDA_inversa : Fcn  Expr=1/(u[1]+c8*u[2])-c9/(1+u[2]^3)
  Mux : Mux  Inputs=2
  Mux1 : Mux  Inputs=2
  Mux2 : Mux  Inputs=2
  Mux3 : Mux  Inputs=3
  calcula_lambda : Fcn  Expr=u[2]*R/u[1]
  parell_turbina : Outport
  Cp : Outport  Port=2
  wires:
  Calcula_parell/1 -> parell_turbina/1
  Mux3/1 -> Calcula_parell/1
  Calcula_Cp/1 -> Cp/1, Mux3/1
  Mux2/1 -> Calcula_Cp/1
  LAMBDA_inversa/1 -> Mux2/1
  Mux/1 -> LAMBDA_inversa/1
  theta_aleps/1 -> Mux2/2, Mux/2
  calcula_lambda/1 -> Mux/1
  velocitat_vent/1 -> Mux3/2, Mux1/1
  omega_aleps/1 -> Mux3/3, Mux1/2
  Mux1/1 -> calcula_lambda/1

== system Non_WindFarm/FOM/Wind Farm/Wind Turbine Strings/String1/WT3/Transformer-complex/homopolar sequence/Park ==
  theta_r : Inport
  Constant4 : Constant  Value=2*pi/3
  Gain7 : Gain  Gain=2/3
  Matrix Concatenate1 : Concatenate  NumInputs=3  Mode=Multidimensional array  ConcatenateDimension=2
  Matrix Concatenate2 : Concatenate  Mode=Multidimensional array  ConcatenateDimension=2
  Mux2 : Mux  Inputs=2
  Mux3 : Mux  Inputs=2
  Mux4 : Mux  Inputs=2
  Mux5 : Mux  Inputs=3
  Mux6 : Mux  Inputs=3
  Sum1 : Sum  Inputs=|++
  Sum2 : Sum  Inputs=|+-
  Trigonometric Function : Trigonometry  Operator=cos
  Trigonometric Function1 : Trigonometry
  Trigonometric Function2 : Trigonometry  Operator=cos
  Trigonometric Function3 : Trigonometry
  Trigonometric Function4 : Trigonometry  Operator=cos
  Trigonometric Function5 : Trigonometry
  Tthetar : Outport
  nTthetar : Outport  Port=2
  wires:
  theta_r/1 -> Sum1/1, Sum2/1, Trigonometric Function/1, Trigonometric Function1/1
  Sum2/1 -> Trigonometric Function2/1, Trigonometric Function3/1
  Sum1/1 -> Trigonometric Function4/1, Trigonometric Function5/1
  Constant4/1 -> Sum2/2, Sum1/2
  Trigonometric Function/1 -> Mux2/1, Mux5/1
  Trigonometric Function1/1 -> Mux2/2, Mux6/1
  Trigonometric Function2/1 -> Mux3/1, Mux5/2
  Trigonometric Function3/1 -> Mux3/2, Mux6/2
  Trigonometric Function4/1 -> Mux4/1, Mux5/3
  Trigonometric Function5/1 -> Mux4/2, Mux6/3
  Mux2/1 -> Matrix Concatenate1/1
  Mux3/1 -> Matrix Concatenate1/2
  Mux4/1 -> Matrix Concatenate1/3
  Matrix Concatenate1/1 -> Gain7/1
  Mux5/1 -> Matrix Concatenate2/1
  Mux6/1 -> Matrix Concatenate2/2
  Gain7/1 -> Tthetar/1
  Matrix Concatenate2/1 -> nTthetar/1

== system Non_WindFarm/FOM/Wind Farm/Wind Turbine Strings/String1/WT3/Transformer-complex/homopolar sequence/homopolar sequence 1 ==
  note: 1/3*v0
  v : Inport
  Add5 : Sum  Inputs=-+
  Constant : Constant  Value=1/3*ones(3)
  Product3 : Product  Multiplication=Matrix(*)  RndMeth=Zero
  v_bar : Outport
  wires:
  Add5/1 -> v_bar/1
  Product3/1 -> Add5/1
  Constant/1 -> Product3/1
  v/1 -> Product3/2, Add5/2

== system Non_WindFarm/FOM/Wind Farm/Wind Turbine Strings/String1/WT3/Transformer-complex/homopolar sequence/homopolar sequence 2 ==
  note: 1/3*v0
  v : Inport
  Add5 : Sum  Inputs=-+
  Constant : Constant  Value=[1/9,1/9,1/9;1/9,1/9,1/9;1/9,1/9,1/9]
  Product3 : Product  Multiplication=Matrix(*)  RndMeth=Zero
  v_bar : Outport
  wires:
  Add5/1 -> v_bar/1
  Product3/1 -> Add5/1
  Constant/1 -> Product3/1
  v/1 -> Product3/2, Add5/2

== system Non_WindFarm/FOM/Wind Farm/Wind Turbine Strings/String1/WT3/WFG/Control Electric Generador/PI ==
  e : Inport
  Demux : Demux  Outputs=2
  Mux2 : Mux  Inputs=2
  Transfer Fcn : TransferFcn  Numerator=[qKp qKi]  Denominator=[1 0]
  Transfer Fcn1 : TransferFcn  Numerator=[dKp dKi]  Denominator=[1 0]
  u : Outport
  wires:
  Mux2/1 -> u/1
  e/1 -> Demux/1
  Demux/2 -> Transfer Fcn1/1
  Demux/1 -> Transfer Fcn/1
  Transfer Fcn1/1 -> Mux2/2
  Transfer Fcn/1 -> Mux2/1

== system Non_WindFarm/FOM/Wind Farm/Wind Turbine Strings/String1/WT3/WFG/Control Electric Generador/Park ==
  theta_r : Inport
  Constant4 : Constant  Value=2*pi/3
  Gain7 : Gain  Gain=2/3
  Matrix Concatenate1 : Concatenate  NumInputs=3  Mode=Multidimensional array  ConcatenateDimension=2
  Matrix Concatenate2 : Concatenate  Mode=Multidimensional array  ConcatenateDimension=2
  Mux2 : Mux  Inputs=2
  Mux3 : Mux  Inputs=2
  Mux4 : Mux  Inputs=2
  Mux5 : Mux  Inputs=3
  Mux6 : Mux  Inputs=3
  Sum1 : Sum  Inputs=|++
  Sum2 : Sum  Inputs=|+-
  Trigonometric Function : Trigonometry  Operator=cos
  Trigonometric Function1 : Trigonometry
  Trigonometric Function2 : Trigonometry  Operator=cos
  Trigonometric Function3 : Trigonometry
  Trigonometric Function4 : Trigonometry  Operator=cos
  Trigonometric Function5 : Trigonometry
  Tthetar : Outport
  nTthetar : Outport  Port=2
  wires:
  Matrix Concatenate2/1 -> nTthetar/1
  Gain7/1 -> Tthetar/1
  Mux6/1 -> Matrix Concatenate2/2
  Mux5/1 -> Matrix Concatenate2/1
  Matrix Concatenate1/1 -> Gain7/1
  Mux4/1 -> Matrix Concatenate1/3
  Mux3/1 -> Matrix Concatenate1/2
  Mux2/1 -> Matrix Concatenate1/1
  Trigonometric Function5/1 -> Mux6/3, Mux4/2
  Trigonometric Function4/1 -> Mux5/3, Mux4/1
  Trigonometric Function3/1 -> Mux6/2, Mux3/2
  Trigonometric Function2/1 -> Mux5/2, Mux3/1
  Trigonometric Function1/1 -> Mux6/1, Mux2/2
  Trigonometric Function/1 -> Mux5/1, Mux2/1
  Constant4/1 -> Sum1/2, Sum2/2
  Sum1/1 -> Trigonometric Function5/1, Trigonometric Function4/1
  Sum2/1 -> Trigonometric Function3/1, Trigonometric Function2/1
  theta_r/1 -> Trigonometric Function1/1, Trigonometric Function/1, Sum2/1, Sum1/1

== system Non_WindFarm/FOM/Wind Farm/Wind Turbine Strings/String1/WT3/WFG/Control Electric Generador/Sat inf ==
  in : Inport
  Abs : Abs  SaturateOnIntegerOverflow=off
  Constant3 : Constant  Value=0.01
  Relational Operator : RelationalOperator  Operator=>  OutDataTypeStr=boolean  InputSameDT=off
  Switch : Switch  Criteria=u2 > Threshold  SaturateOnIntegerOverflow=off  InputSameDT=off
  out : Outport
  wires:
  Switch/1 -> out/1
  in/1 -> Switch/1, Abs/1
  Relational Operator/1 -> Switch/2
  Constant3/1 -> Switch/3, Relational Operator/2
  Abs/1 -> Relational Operator/1

== system Non_WindFarm/FOM/Wind Farm/Wind Turbine Strings/String1/WT3/WFG/Control de Corrent de Xarxa2/PI_d ==
  e : Inport
  Demux : Demux  Outputs=2
  Mux2 : Mux  Inputs=2
  Transfer Fcn : TransferFcn  Numerator=[Kp Ki]  Denominator=[1,0]
  Transfer Fcn1 : TransferFcn  Numerator=[Kp Ki]  Denominator=[1,0]
  u : Outport
  wires:
  Mux2/1 -> u/1
  e/1 -> Demux/1
  Demux/2 -> Transfer Fcn1/1
  Demux/1 -> Transfer Fcn/1
  Transfer Fcn1/1 -> Mux2/2
  Transfer Fcn/1 -> Mux2/1

== system Non_WindFarm/FOM/Wind Farm/Wind Turbine Strings/String1/WT3/WFG/Control de Corrent de Xarxa2/rotacio1 ==
  theta : Inport
  Constant1 : Constant  Value=2*pi/3
  Gain1 : Gain  Gain=-1
  Matrix Concatenate1 : Concatenate  Mode=Multidimensional array  ConcatenateDimension=2
  Matrix Concatenate2 : Concatenate  Mode=Multidimensional array  ConcatenateDimension=2
  Mux1 : Mux  Inputs=3
  Mux2 : Mux  Inputs=2
  Mux3 : Mux  Inputs=2
  Mux5 : Mux  Inputs=3
  Sum4 : Sum  Inputs=|+-
  Sum5 : Sum  Inputs=|++
  Sum6 : Sum  Inputs=|+-
  Sum7 : Sum  Inputs=|++
  Trigonometric Function{,6,8,10} (4 alike) : Trigonometry  Operator=cos
  Trigonometric Function{1,7,9,11} (4 alike) : Trigonometry
  T : Outport
  nT : Outport  Port=2
  wires:
  Gain1/1 -> Mux3/1
  Mux1/1 -> Matrix Concatenate2/2
  Mux5/1 -> Matrix Concatenate2/1
  Trigonometric Function11/1 -> Mux1/3
  Trigonometric Function7/1 -> Mux1/2
  Trigonometric Function9/1 -> Mux1/1
  Trigonometric Function8/1 -> Mux5/3
  Trigonometric Function10/1 -> Mux5/2
  Trigonometric Function6/1 -> Mux5/1
  Sum7/1 -> Trigonometric Function11/1
  Sum6/1 -> Trigonometric Function7/1
  Sum5/1 -> Trigonometric Function8/1
  Constant1/1 -> Sum7/2, Sum6/2, Sum5/2, Sum4/2
  Sum4/1 -> Trigonometric Function10/1
  theta/1 -> Trigonometric Function1/1, Trigonometric Function/1, Sum7/1, Sum6/1, Trigonometric Function9/1, Sum5/1, Sum4/1, Trigonometric Function6/1
  Matrix Concatenate2/1 -> nT/1
  Matrix Concatenate1/1 -> T/1
  Mux3/1 -> Matrix Concatenate1/2
  Mux2/1 -> Matrix Concatenate1/1
  Trigonometric Function1/1 -> Mux2/2, Gain1/1
  Trigonometric Function/1 -> Mux3/2, Mux2/1

== system Non_WindFarm/FOM/Wind Farm/Wind Turbine Strings/String1/WT3/WFG/Maquina Sincrona/Park ==
  note: Page 24 eq 3.12
  theta_r : Inport
  Constant4 : Constant  Value=2*pi/3
  Gain7 : Gain  Gain=2/3
  Matrix Concatenate1 : Concatenate  NumInputs=3  Mode=Multidimensional array  ConcatenateDimension=2
  Matrix Concatenate2 : Concatenate  Mode=Multidimensional array  ConcatenateDimension=2
  Mux2 : Mux  Inputs=2
  Mux3 : Mux  Inputs=2
  Mux4 : Mux  Inputs=2
  Mux5 : Mux  Inputs=3
  Mux6 : Mux  Inputs=3
  Sum1 : Sum  Inputs=|++
  Sum2 : Sum  Inputs=|+-
  Trigonometric Function : Trigonometry  Operator=cos
  Trigonometric Function1 : Trigonometry
  Trigonometric Function2 : Trigonometry  Operator=cos
  Trigonometric Function3 : Trigonometry
  Trigonometric Function4 : Trigonometry  Operator=cos
  Trigonometric Function5 : Trigonometry
  Tthetar : Outport
  nTthetar : Outport  Port=2
  wires:
  Sum1/1 -> Trigonometric Function4/1, Trigonometric Function5/1
  Sum2/1 -> Trigonometric Function2/1, Trigonometric Function3/1
  theta_r/1 -> Trigonometric Function/1, Trigonometric Function1/1, Sum2/1, Sum1/1
  Matrix Concatenate2/1 -> nTthetar/1
  Gain7/1 -> Tthetar/1
  Mux6/1 -> Matrix Concatenate2/2
  Mux5/1 -> Matrix Concatenate2/1
  Matrix Concatenate1/1 -> Gain7/1
  Mux4/1 -> Matrix Concatenate1/3
  Mux3/1 -> Matrix Concatenate1/2
  Mux2/1 -> Matrix Concatenate1/1
  Trigonometric Function5/1 -> Mux6/3, Mux4/2
  Trigonometric Function4/1 -> Mux5/3, Mux4/1
  Trigonometric Function3/1 -> Mux6/2, Mux3/2
  Trigonometric Function2/1 -> Mux5/2, Mux3/1
  Trigonometric Function1/1 -> Mux6/1, Mux2/2
  Trigonometric Function/1 -> Mux5/1, Mux2/1
  Constant4/1 -> Sum1/2, Sum2/2

== system Non_WindFarm/FOM/Wind Farm/Wind Turbine Strings/String1/WT3/WFG/Mecanica nolineal i vent/Turbina ==
  note: Beta-pitch angle
  note: Vw-wind speed
  note: Wt-turbine speed
  note: Gamma_t-Wind turbine torque
  note: Page 8
  velocitat_vent : Inport
  omega_aleps : Inport  Port=2
  theta_aleps : Inport  Port=3
  Calcula_Cp : Fcn  Expr=c1*(c2*u[1]-c3*u[2]-c4*u[2]^c5-c6)*exp(-c7*u[1])
  Calcula_parell : Fcn  Expr=u[1]*rho*A*u[2]^3/(2*u[3])
  LAMBDA_inversa : Fcn  Expr=1/(u[1]+c8*u[2])-c9/(1+u[2]^3)
  Mux : Mux  Inputs=2
  Mux1 : Mux  Inputs=2
  Mux2 : Mux  Inputs=2
  Mux3 : Mux  Inputs=3
  calcula_lambda : Fcn  Expr=u[2]*R/u[1]
  parell_turbina : Outport
  Cp : Outport  Port=2
  wires:
  Calcula_parell/1 -> parell_turbina/1
  Mux3/1 -> Calcula_parell/1
  Calcula_Cp/1 -> Cp/1, Mux3/1
  Mux2/1 -> Calcula_Cp/1
  LAMBDA_inversa/1 -> Mux2/1
  Mux/1 -> LAMBDA_inversa/1
  theta_aleps/1 -> Mux2/2, Mux/2
  calcula_lambda/1 -> Mux/1
  velocitat_vent/1 -> Mux3/2, Mux1/1
  omega_aleps/1 -> Mux3/3, Mux1/2
  Mux1/1 -> calcula_lambda/1

== system Non_WindFarm/FOM/Wind Farm/Wind Turbine Strings/String1/WT4/Transformer-complex/homopolar sequence/Park ==
  theta_r : Inport
  Constant4 : Constant  Value=2*pi/3
  Gain7 : Gain  Gain=2/3
  Matrix Concatenate1 : Concatenate  NumInputs=3  Mode=Multidimensional array  ConcatenateDimension=2
  Matrix Concatenate2 : Concatenate  Mode=Multidimensional array  ConcatenateDimension=2
  Mux2 : Mux  Inputs=2
  Mux3 : Mux  Inputs=2
  Mux4 : Mux  Inputs=2
  Mux5 : Mux  Inputs=3
  Mux6 : Mux  Inputs=3
  Sum1 : Sum  Inputs=|++
  Sum2 : Sum  Inputs=|+-
  Trigonometric Function : Trigonometry  Operator=cos
  Trigonometric Function1 : Trigonometry
  Trigonometric Function2 : Trigonometry  Operator=cos
  Trigonometric Function3 : Trigonometry
  Trigonometric Function4 : Trigonometry  Operator=cos
  Trigonometric Function5 : Trigonometry
  Tthetar : Outport
  nTthetar : Outport  Port=2
  wires:
  Matrix Concatenate2/1 -> nTthetar/1
  Gain7/1 -> Tthetar/1
  Mux6/1 -> Matrix Concatenate2/2
  Mux5/1 -> Matrix Concatenate2/1
  Matrix Concatenate1/1 -> Gain7/1
  Mux4/1 -> Matrix Concatenate1/3
  Mux3/1 -> Matrix Concatenate1/2
  Mux2/1 -> Matrix Concatenate1/1
  Trigonometric Function5/1 -> Mux6/3, Mux4/2
  Trigonometric Function4/1 -> Mux5/3, Mux4/1
  Trigonometric Function3/1 -> Mux6/2, Mux3/2
  Trigonometric Function2/1 -> Mux5/2, Mux3/1
  Trigonometric Function1/1 -> Mux6/1, Mux2/2
  Trigonometric Function/1 -> Mux5/1, Mux2/1
  Constant4/1 -> Sum1/2, Sum2/2
  Sum1/1 -> Trigonometric Function5/1, Trigonometric Function4/1
  Sum2/1 -> Trigonometric Function3/1, Trigonometric Function2/1
  theta_r/1 -> Trigonometric Function1/1, Trigonometric Function/1, Sum2/1, Sum1/1

== system Non_WindFarm/FOM/Wind Farm/Wind Turbine Strings/String1/WT4/Transformer-complex/homopolar sequence/homopolar sequence 1 ==
  note: 1/3*v0
  v : Inport
  Add5 : Sum  Inputs=-+
  Constant : Constant  Value=1/3*ones(3)
  Product3 : Product  Multiplication=Matrix(*)  RndMeth=Zero
  v_bar : Outport
  wires:
  v/1 -> Add5/2, Product3/2
  Constant/1 -> Product3/1
  Product3/1 -> Add5/1
  Add5/1 -> v_bar/1

== system Non_WindFarm/FOM/Wind Farm/Wind Turbine Strings/String1/WT4/Transformer-complex/homopolar sequence/homopolar sequence 2 ==
  note: 1/3*v0
  v : Inport
  Add5 : Sum  Inputs=-+
  Constant : Constant  Value=[1/9,1/9,1/9;1/9,1/9,1/9;1/9,1/9,1/9]
  Product3 : Product  Multiplication=Matrix(*)  RndMeth=Zero
  v_bar : Outport
  wires:
  v/1 -> Add5/2, Product3/2
  Constant/1 -> Product3/1
  Product3/1 -> Add5/1
  Add5/1 -> v_bar/1

== system Non_WindFarm/FOM/Wind Farm/Wind Turbine Strings/String1/WT4/WFG/Control Electric Generador/PI ==
  e : Inport
  Demux : Demux  Outputs=2
  Mux2 : Mux  Inputs=2
  Transfer Fcn : TransferFcn  Numerator=[qKp qKi]  Denominator=[1 0]
  Transfer Fcn1 : TransferFcn  Numerator=[dKp dKi]  Denominator=[1 0]
  u : Outport
  wires:
  Mux2/1 -> u/1
  e/1 -> Demux/1
  Demux/2 -> Transfer Fcn1/1
  Demux/1 -> Transfer Fcn/1
  Transfer Fcn1/1 -> Mux2/2
  Transfer Fcn/1 -> Mux2/1
